simulink model "DraftSimpleEstimator_R2021b"  (R2021b)
settings: Solver=ode1  StartTime=0.0  StopTime=inf  FixedStep=10e-3  RelTol=1e-3
libraries: TcTargetLib x11
settings Model: Creator=Mergin  LastModifiedBy=ATLabor
settings OptimizationCC: DefaultParameterBehavior=Inlined  LocalBlockOutputs=off
settings DebuggingCC: UnconnectedInputMsg=none  UnconnectedOutputMsg=none  UnconnectedLineMsg=none
settings ModelReferenceCC: EnableRefExpFcnMdlSchedulingChecks=off
settings RTWCC: Description=TwinCAT GRT Target  SystemTargetFile=TwinCatGrt.tlc  GenCodeOnly=on  TemplateMakefile=tcgrt_msbuild.tmf  TargetLang=C++  DLArmComputeVersion=20.02.1
settings STFCustomTargetCC: TargetLangStandard=C++11 (ISO)  CombineOutputUpdateFcns=on  CodeInterfacePackaging=Reusable function  CPPClassGenCompliant=on  GRTInterface=off  GenerateAllocFcn=on  SystemTargetFile=TwinCatGrt.tlc
settings GRTTargetCC: TargetLangStandard=C++11 (ISO)  ParMdlRefBuildCompliant=off  CompOptLevelCompliant=off  ConcurrentExecutionCompliant=off  MatFileLogging=off  CodeInterfacePackaging=Reusable function  GenerateAllocFcn=on  UseToolchainInfoCompliant=off  ExtModeMexFile=TcExtModeClient

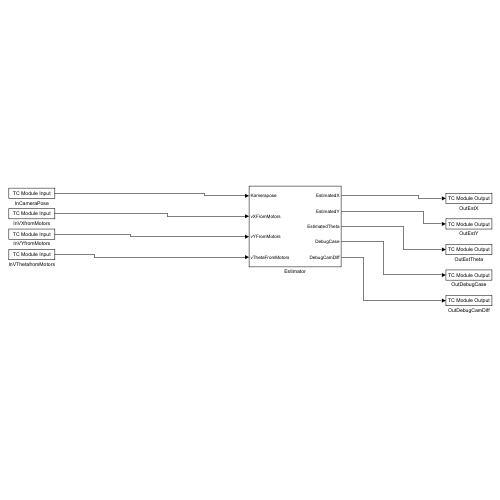
[thumbnail: Simulink's stored preview of the top-level diagram]
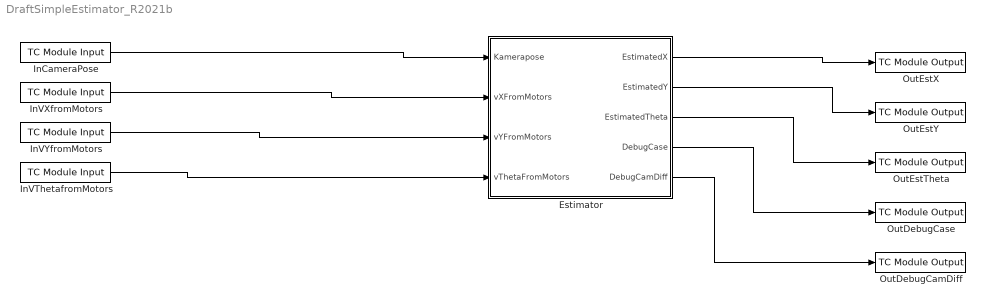
== system DraftSimpleEstimator_R2021b ==
  Estimator : Subsystem
  InCameraPose : TcTargetLib/TC Module Input  PortDataType=double  PortDim=3  Value=[0 0 0]  SampleTime=-1  CodeGenConnectType=DataArea (InputDst)  DataTypeOverride=on
      settings: SourceProductName=Beckhoff TwinCAT Target
  InVThetafromMotors : TcTargetLib/TC Module Input  PortDataType=double  PortDim=1  Value=0  SampleTime=-1  CodeGenConnectType=DataArea (InputDst)  DataTypeOverride=off
      settings: SourceProductName=Beckhoff TwinCAT Target
  InVXfromMotors : TcTargetLib/TC Module Input  PortDataType=double  PortDim=1  Value=0  SampleTime=-1  CodeGenConnectType=DataArea (InputDst)  DataTypeOverride=off
      settings: SourceProductName=Beckhoff TwinCAT Target
  InVYfromMotors : TcTargetLib/TC Module Input  PortDataType=double  PortDim=1  Value=0  SampleTime=-1  CodeGenConnectType=DataArea (InputDst)  DataTypeOverride=off
      settings: SourceProductName=Beckhoff TwinCAT Target
  OutDebugCamDiff : TcTargetLib/TC Module Output  PortDataType=double  PortDim=1  SampleTime=-1  CodeGenConnectType=DataArea (OutputSrc)  DataTypeOverride=off
      settings: SourceProductName=Beckhoff TwinCAT Target
  OutDebugCase : TcTargetLib/TC Module Output  PortDataType=double  PortDim=1  SampleTime=-1  CodeGenConnectType=DataArea (OutputSrc)  DataTypeOverride=off
      settings: SourceProductName=Beckhoff TwinCAT Target
  OutEstTheta : TcTargetLib/TC Module Output  PortDataType=double  PortDim=1  SampleTime=-1  CodeGenConnectType=DataArea (OutputSrc)  DataTypeOverride=off
      settings: SourceProductName=Beckhoff TwinCAT Target
  OutEstX : TcTargetLib/TC Module Output  PortDataType=double  PortDim=1  SampleTime=-1  CodeGenConnectType=DataArea (OutputSrc)  DataTypeOverride=off
      settings: SourceProductName=Beckhoff TwinCAT Target
  OutEstY : TcTargetLib/TC Module Output  PortDataType=double  PortDim=1  SampleTime=-1  CodeGenConnectType=DataArea (OutputSrc)  DataTypeOverride=off
      settings: SourceProductName=Beckhoff TwinCAT Target
  wires:
  InCameraPose/1 -> Estimator/1(Kamerapose)
  InVXfromMotors/1 -> Estimator/2(vXFromMotors)
  InVYfromMotors/1 -> Estimator/3(vYFromMotors)
  InVThetafromMotors/1 -> Estimator/4(vThetaFromMotors)
  Estimator/1(EstimatedX) -> OutEstX/1
  Estimator/2(EstimatedY) -> OutEstY/1
  Estimator/3(EstimatedTheta) -> OutEstTheta/1
  Estimator/4(DebugCase) -> OutDebugCase/1
  Estimator/5(DebugCamDiff) -> OutDebugCamDiff/1

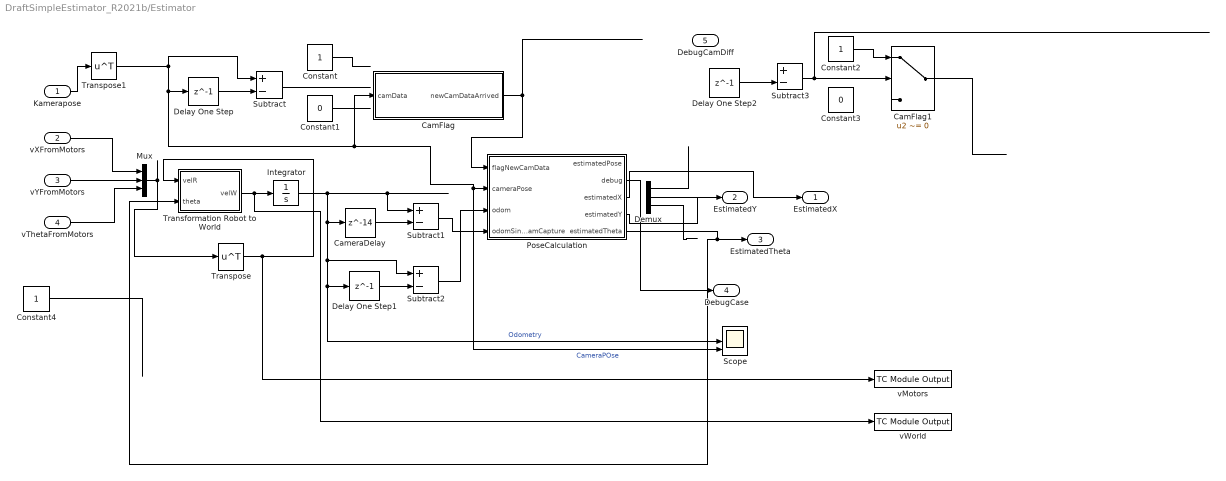
== system DraftSimpleEstimator_R2021b/Estimator ==
  Kamerapose : Inport
  vXFromMotors : Inport  Port=2
  vYFromMotors : Inport  Port=3
  vThetaFromMotors : Inport  Port=4
  CamFlag : MATLAB Function  TreatAsAtomicUnit=on
  CamFlag1 : Switch  Criteria=u2 ~= 0
  CameraDelay : Delay  DelayLength=14
  Constant : Constant
  Constant1 : Constant  Value=0
  Constant2 : Constant
  Constant3 : Constant  Value=0
  Constant4 : Constant
  Delay One Step : Delay  DelayLength=1
  Delay One Step1 : Delay  DelayLength=1
  Delay One Step2 : Delay  DelayLength=1
  Demux : Demux  Outputs=3
  Integrator : Integrator
  Mux : Mux  Inputs=3
  PoseCalculation : MATLAB Function  TreatAsAtomicUnit=on
  Scope : Scope  NumInputPorts=3
  Subtract{,1..3} (4 alike) : Sum  Inputs=+-
  Transformation Robot to World : MATLAB Function  TreatAsAtomicUnit=on
  Transpose : Math  Operator=transpose  SaturateOnIntegerOverflow=on
  Transpose1 : Math  Operator=transpose  SaturateOnIntegerOverflow=on
  vMotors : TcTargetLib/TC Module Output  PortDataType=double  PortDim=3  SampleTime=-1  CodeGenConnectType=DataArea (OutputSrc)  DataTypeOverride=off
      settings: SourceProductName=Beckhoff TwinCAT Target
  vWorld : TcTargetLib/TC Module Output  PortDataType=double  PortDim=3  SampleTime=-1  CodeGenConnectType=DataArea (OutputSrc)  DataTypeOverride=off
      settings: SourceProductName=Beckhoff TwinCAT Target
  EstimatedX : Outport
  EstimatedY : Outport  Port=2
  EstimatedTheta : Outport  Port=3
  DebugCase : Outport  Port=4
  DebugCamDiff : Outport  Port=5
  wires:
  Demux/1 -> ?
  Constant/1 -> ?
  Delay One Step/1 -> Subtract/2
  Demux/2 -> ?
  vThetaFromMotors/1 -> Mux/3
  Subtract1/1 -> PoseCalculation/4(odomSinceCamCapture)
  Mux/1 -> Transpose/1
  CameraDelay/1 -> Subtract1/2
  Constant1/1 -> ?
  Transformation Robot to World/1(velW) -> vWorld/1, Integrator/1
  vXFromMotors/1 -> Mux/1
  Transpose1/1 -> Scope/3, PoseCalculation/2(cameraPose), CamFlag/1(camData), Delay One Step/1, Subtract/1  "CameraPOse"
  Integrator/1 -> Subtract1/1, Delay One Step1/1, Scope/2, Subtract2/1, CameraDelay/1  "Odometry"
  vYFromMotors/1 -> Mux/2
  CamFlag/1(newCamDataArrived) -> PoseCalculation/1(flagNewCamData)
  ? -> Scope/1, Demux/1
  Subtract/1 -> ?
  Kamerapose/1 -> Transpose1/1
  Delay One Step1/1 -> Subtract2/2
  Subtract2/1 -> PoseCalculation/3(odom)
  PoseCalculation/2(debug) -> DebugCase/1
  Constant2/1 -> CamFlag1/1
  CamFlag1/1 -> ?
  Subtract3/1 -> CamFlag1/2
  ? -> Subtract3/1  "CameraPOse"
  Delay One Step2/1 -> Subtract3/2
  Transpose/1 -> vMotors/1, Transformation Robot to World/1(velR)
  Demux/3 -> ?
  PoseCalculation/4(estimatedY) -> EstimatedY/1
  PoseCalculation/3(estimatedX) -> EstimatedX/1
  Constant4/1 -> ?
  PoseCalculation/5(estimatedTheta) -> Transformation Robot to World/2(theta), EstimatedTheta/1

== matlab function DraftSimpleEstimator_R2021b/Estimator/PoseCalculation ==
  settings: updateMethod=DISCRETE
  data: flagNewCamData input; cameraPose input; estimatedPose output; odom input; odomSinceCamCapture input; debug output; estimatedX output; estimatedY output; estimatedTheta output
function [estimatedPose, debug, estimatedX, estimatedY, estimatedTheta]= fcn(flagNewCamData, cameraPose, odom, odomSinceCamCapture)

% Variables
persistent estPoseOld

if isempty(estPoseOld)
    estPoseOld = [0 0 0];
end

    % Case 1: Camera Flag is set (New Cameradata) and CameraData is valid
if flagNewCamData == 1
    estimatedPose = cameraPose(1:3) + odomSinceCamCapture;   %OdomSinceCamCapture describes the pose changes since the camera captured the position because the camera data is delayed. in this time the robot drives further.
    estPoseOld = estimatedPose;
    debug = 1;

    % Case 2: No new Cameradata or invalid Cmeradata (integrate transformed velocities of
    % roboter in worldframe
else
    estimatedPose = estPoseOld + odom;
    estPoseOld = estimatedPose;
    debug =2;
end

estimatedX = estimatedPose(1);
estimatedY = estimatedPose(2);
estimatedTheta = estimatedPose(3);

== matlab function DraftSimpleEstimator_R2021b/Estimator/Transformation Robot to World ==
  data: velR input; velW output size=[1 3]; theta input
function velW = fcn(velR, theta)
    TMat = [cos(theta)    -sin(theta)   0;
            sin(theta)    cos(theta)    0;
            0             0             1];
    velW = velR*transpose(TMat);
end

== matlab function DraftSimpleEstimator_R2021b/Estimator/CamFlag ==
  data: camData input; newCamDataArrived output
function newCamDataArrived = fcn(camData)

persistent oldCamData

if isempty(oldCamData)
    oldCamData = [0 0 0];
end

if camData ~= oldCamData
    newCamDataArrived = true;
else
    newCamDataArrived = false;
    oldCamData = camData;
end
